simulink library "fauTurbComponent_ul"  (R2022a)
settings: Solver=VariableStepAuto  StartTime=0.0  StopTime=10.0  RelTol=1e-3
undefined symbols (not defined in the file): env
settings Model: Creator=mcobb  LastModifiedBy=lhill8
settings SolverCC: AlgebraicLoopSolver=TrustRegion
settings DebuggingCC: UnconnectedInputMsg=warning  UnconnectedOutputMsg=warning  UnconnectedLineMsg=warning  SFMachineParentedDataDiag=warning  ArithmeticOperatorsInVariantConditions=warning
settings SFSimCC: CustomCodeUndefinedFunction=UseInterfaceOnly

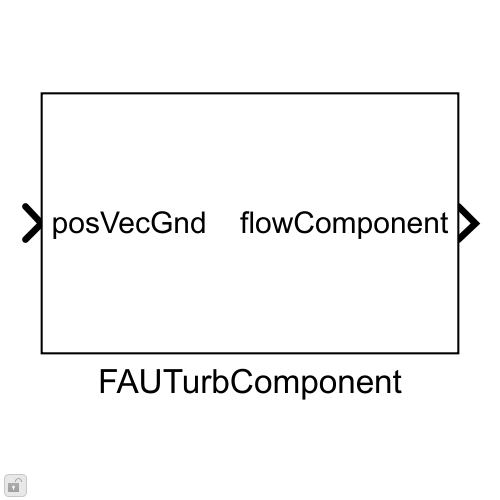
[thumbnail: Simulink's stored preview of the top-level diagram]
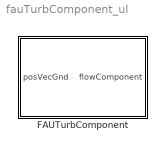
== system fauTurbComponent_ul ==
  FAUTurbComponent : Subsystem

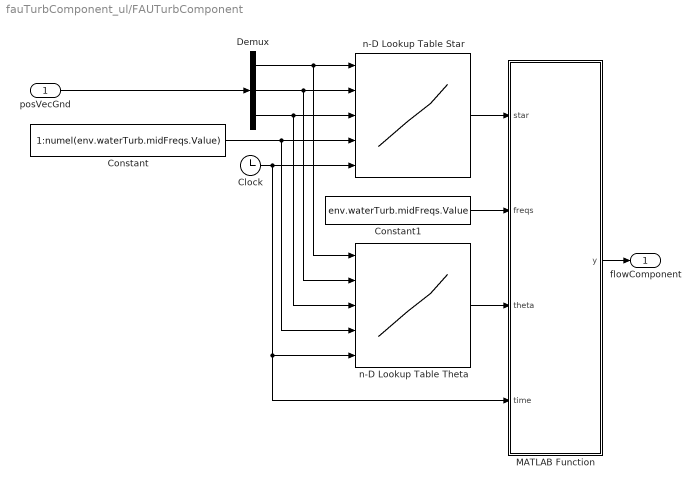
== system fauTurbComponent_ul/FAUTurbComponent ==
  posVecGnd : Inport
  Clock : Clock
  Constant : Constant  Value=1:numel(env.waterTurb.midFreqs.Value)
  Constant1 : Constant  Value=env.waterTurb.midFreqs.Value
  Demux : Demux  Outputs=3
  MATLAB Function : MATLAB Function  TreatAsAtomicUnit=on
  n-D Lookup Table Star : Lookup_n-D  NumberOfTableDimensions=5  LookupTableObject=x  BreakpointsForDimension1=env.waterTurb.uStarLUT.Value.Breakpoints(1).Value  BreakpointsForDimension2=env.waterTurb.uStarLUT.Value.Breakpoints(2).Value  BreakpointsForDimension3=env.waterTurb.uStarLUT.Value.Breakpoints(3).Value  BreakpointsForDimension4=env.waterTurb.uStarLUT.Value.Breakpoints(4).Value  BreakpointsForDimension5=env.waterTurb.uStarLUT.Value.Breakpoints(5).Value  Table=env.waterTurb.uStarLUT.Value.Table.Value  InternalRulePriority=Speed  RndMeth=Simplest
      settings: InputPortMap=u0,u1,u2,u3,u4
  n-D Lookup Table Theta : Lookup_n-D  NumberOfTableDimensions=5  LookupTableObject=x  BreakpointsForDimension1=env.waterTurb.uThLUT.Value.Breakpoints(1).Value  BreakpointsForDimension2=env.waterTurb.uThLUT.Value.Breakpoints(2).Value  BreakpointsForDimension3=env.waterTurb.uThLUT.Value.Breakpoints(3).Value  BreakpointsForDimension4=env.waterTurb.uThLUT.Value.Breakpoints(4).Value  BreakpointsForDimension5=env.waterTurb.uThLUT.Value.Breakpoints(5).Value  Table=env.waterTurb.uThLUT.Value.Table.Value  InternalRulePriority=Speed  RndMeth=Simplest
      settings: InputPortMap=u0,u1,u2,u3,u4
  flowComponent : Outport  VectorParamsAs1DForOutWhenUnconnected=off
  wires:
  Demux/2 -> n-D Lookup Table Theta/2, n-D Lookup Table Star/2
  Demux/1 -> n-D Lookup Table Theta/1, n-D Lookup Table Star/1
  Demux/3 -> n-D Lookup Table Theta/3, n-D Lookup Table Star/3
  posVecGnd/1 -> Demux/1
  Constant/1 -> n-D Lookup Table Theta/4, n-D Lookup Table Star/4
  Clock/1 -> n-D Lookup Table Theta/5, MATLAB Function/4(time), n-D Lookup Table Star/5
  n-D Lookup Table Star/1 -> MATLAB Function/1(star)
  n-D Lookup Table Theta/1 -> MATLAB Function/3(theta)
  MATLAB Function/1(y) -> flowComponent/1
  Constant1/1 -> MATLAB Function/2(freqs)

== matlab function fauTurbComponent_ul/FAUTurbComponent/MATLAB Function ==
  data: star input; freqs input; y output; theta input; time input
function y = fcn(star,freqs,theta,time)
y = sum(abs(star(:)).*sin(2*pi*freqs(:)*time+theta(:)));
